simulink model "dynamics_kinematics_subsystem"  (R2025a)
settings: Solver=VariableStepAuto  StartTime=0.0  StopTime=10.0  RelTol=1e-3
undefined symbols (not defined in the file or in its folder): IC, Sat
libraries: aerolibutil x2, matrix_library x1, sharedutil x1
settings Model: Creator=arroy  LastModifiedBy=arroy

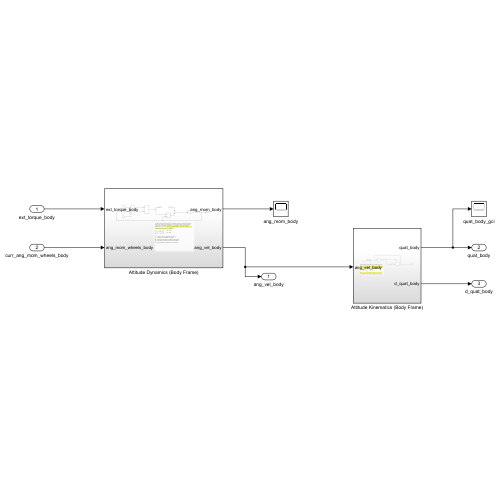
[thumbnail: Simulink's stored preview of the top-level diagram]
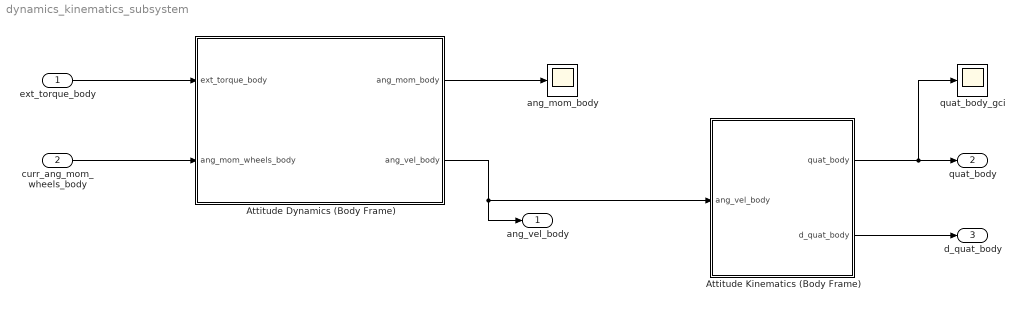
== system dynamics_kinematics_subsystem ==
  ext_torque_body : Inport
  curr_ang_mom_wheels_body : Inport  Port=2
  Attitude Dynamics (Body Frame) : Subsystem
  Attitude Kinematics (Body Frame) : Subsystem
  ang_mom_body : Scope
      settings: ActiveDisplayYMinimum=-0.00017  ActiveDisplayYMaximum=0.00014  DataLoggingVariableName=ScopeData3
  quat_body_gci : Scope
      settings: ActiveDisplayYMinimum=-0.52819  ActiveDisplayYMaximum=1.1698  DataLoggingVariableName=ScopeData5
  ang_vel_body : Outport
  quat_body : Outport  Port=2
  d_quat_body : Outport  Port=3
  wires:
  Attitude Dynamics (Body Frame)/2(ang_vel_body) -> ang_vel_body/1, Attitude Kinematics (Body Frame)/1(ang_vel_body)
  Attitude Kinematics (Body Frame)/1(quat_body) -> quat_body_gci/1, quat_body/1
  ext_torque_body/1 -> Attitude Dynamics (Body Frame)/1(ext_torque_body)
  Attitude Dynamics (Body Frame)/1(ang_mom_body) -> ang_mom_body/1
  curr_ang_mom_wheels_body/1 -> Attitude Dynamics (Body Frame)/2(ang_mom_wheels_body)
  Attitude Kinematics (Body Frame)/2(d_quat_body) -> d_quat_body/1

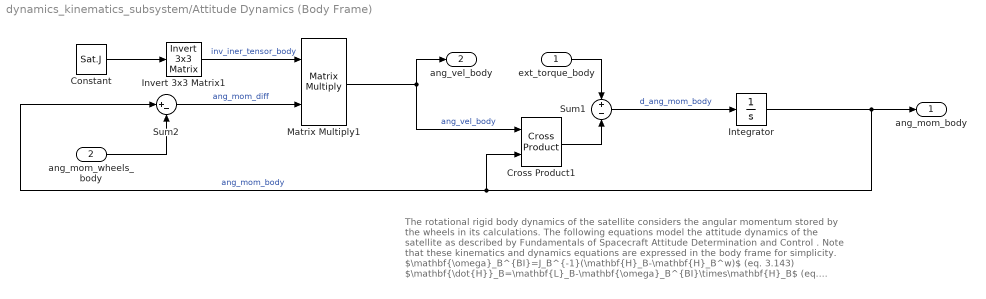
== system dynamics_kinematics_subsystem/Attitude Dynamics (Body Frame) ==
  note: The rotational rigid body dynamics of the satellite considers the angular momentum stored by the wheels in its calculations. The following equations model the attitude dynamics of the satellite as described by Fundamentals of Spacecraft Attitude Determination and Control . Note that these kinematics and dynamics equations are expressed in the body frame for simplicity.
      |
      | $\mathbf{\omega}_B^{BI}=J_B^{-1}(\mathbf{H}_B-\mathbf{H}_B^w)$ (eq. 3.143)
      | $\mathbf{\dot{H}}_B=\mathbf{L}_B-\mathbf{\omega}_B^{BI}\times\mathbf{H}_B$ (eq. 3.80)
      |
      | $\mathbf{\omega}_B^{BI}$ - angular velocity of satellite in body frame
      | $J_B$ - inertia tensor of satellite in body frame
      | $\mathbf{H}_B$ - total angular momentum of satellite in body frame
      | $\mathbf{H}_B^w$ - total angular momentum of wheels in body frame
      | $\mathbf{L}_B$ - moment applied to spacecraft in the body frame
  ext_torque_body : Inport
  ang_mom_wheels_body : Inport  Port=2
  Constant : Constant  Value=Sat.J
  Cross Product1 : matrix_library/Cross Product
  Integrator : Integrator  InitialCondition=IC.w0
  Invert 3x3 Matrix1 : aerolibutil/Invert  3x3 Matrix
  Matrix Multiply1 : Product  Multiplication=Matrix(*)
  Sum1 : Sum  Inputs=+-
  Sum2 : Sum  Inputs=|+-
  ang_mom_body : Outport
  ang_vel_body : Outport  Port=2
  wires:
  Invert 3x3 Matrix1/1 -> Matrix Multiply1/1  "inv_iner_tensor_body"
  Constant/1 -> Invert 3x3 Matrix1/1
  ang_mom_wheels_body/1 -> Sum2/2
  Integrator/1 -> Sum2/1, Cross Product1/2, ang_mom_body/1  "ang_mom_body"
  Matrix Multiply1/1 -> Cross Product1/1, ang_vel_body/1  "ang_vel_body"
  Sum2/1 -> Matrix Multiply1/2  "ang_mom_diff"
  Sum1/1 -> Integrator/1  "d_ang_mom_body"
  ext_torque_body/1 -> Sum1/1
  Cross Product1/1 -> Sum1/2

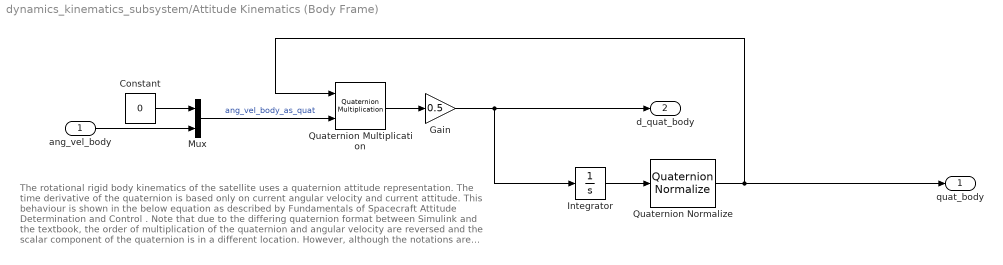
== system dynamics_kinematics_subsystem/Attitude Kinematics (Body Frame) ==
  note: The rotational rigid body kinematics of the satellite uses a quaternion attitude representation. The time derivative of the quaternion is based only on current angular velocity and current attitude. This behaviour is shown in the below equation as described by Fundamentals of Spacecraft Attitude Determination and Control . Note that due to the differing quaternion format between Simulink and the textbook, the order of multiplication of the quaternion and angular velocity are reversed and the scalar component of the quaternion is in a different location. However, although the notations are different, they are functionally the same.
      |
      | $\mathbf{\dot{q}}_{BI}=\frac{1}{2}\mathbf{q}_{BI}\cdot\mathbf{\omega}_B^{BI}=\frac{1}{2}\mathbf{q}_{BI}\cdot\left[\matrix{0 \cr \mathbf{\omega}_B^{BI}}\right]$ (eq. 3.79d)
      |
      | Note that in the above equation, multiplication between a quaternion and vector requires transforming the vector to a quaternion with scalar component of 0, as seen on the RHS.
      |
      | $\mathbf{q}_{BI}$ - current attitude of the spacecraft (rotation from inertial frame to body frame as specified in the inertial frame)
      | $\mathbf{\omega}_{B}^{BI}$ - angular velocity of satellite in body frame
  ang_vel_body : Inport
  Constant : Constant  Value=0
  Gain : Gain  Gain=0.5
  Integrator : Integrator  InitialCondition=IC.q0
  Mux : Mux  Inputs=2
  Quaternion Multiplication : aerolibutil/Quaternion Multiplication
  Quaternion Normalize : sharedutil/Quaternion Normalize  aMode=aMode
  quat_body : Outport  PortDimensions=4
  d_quat_body : Outport  Port=2  PortDimensions=4
  wires:
  Constant/1 -> Mux/1
  ang_vel_body/1 -> Mux/2
  Quaternion Multiplication/1 -> Gain/1
  Mux/1 -> Quaternion Multiplication/2  "ang_vel_body_as_quat"
  Integrator/1 -> Quaternion Normalize/1
  Gain/1 -> d_quat_body/1, Integrator/1
  Quaternion Normalize/1 -> quat_body/1, Quaternion Multiplication/1
